simulink model "CompControl_V2"  (R2025b)
settings: Solver=ode45  StartTime=0.0  StopTime=t_f_cc  RelTol=1e-3
values from neighbouring files (symbols this model uses):
  dh_base = dh_raw    [CompControlTest_V2.m]    (also in NewRun.m)
  dq0_cc = zeros(length(joint_types), 1)    [CompControlTest_V2.m]    (also in NewRun.m = dq0)
  g0 = [0, 0, -9.81]    [CompControlTest_V2.m]    (also in EOMtestCode.m = [0 0 -9.81]; NewRun.m = input_ui.gValues; run.m = [0 0 -9.81]; test.m = input.g0)
  h_e = repmat(h_e', length(t), 1)    [CompControlTest_V2.m]    (also in NewRun.m)
  I_l = params.I_l(:)    [CompControlTest_V2.m]    (also in EOMtestCode.m = [IL1 IL2]; NewRun.m = I_l(:); run.m = sym('I_l', [N 1]); test.m = sym('I_l', [N 1]))
  I_m = params.I_m(:)    [CompControlTest_V2.m]    (also in EOMtestCode.m = [IM1 IM2]; NewRun.m = I_m(:); run.m = sym('I_m', [N 1]); test.m = sym('I_m', [N 1]))
  jt = zeros(N, 1)    [CompControlTest_V2.m]    (also in NewRun.m = zeros(DOF, 1))
  k_r = params.k_r(:)    [CompControlTest_V2.m]    (also in EOMtestCode.m = [kr1; kr2]; NewRun.m = k_r(:); run.m = sym('k_r', [N 1]); test.m = sym('k_r', [N 1]))
  KD = diag([ 45,  45,  45,  18,  18,  18])    [CompControlTest_V2.m]    (also in NewRun.m = eye(6)*K_d)
  KP = diag([500, 500, 500,  80,  80,  80])    [CompControlTest_V2.m]    (also in NewRun.m = eye(6)*K_p)
  m_l = params.m_l(:)    [CompControlTest_V2.m]    (also in EOMtestCode.m = [m1 m2]; NewRun.m = m_l(:); run.m = sym('m_l', [N 1]); test.m = sym('m_l', [N 1]))
  m_m = params.m_m(:)    [CompControlTest_V2.m]    (also in EOMtestCode.m = [mm1 mm2]; NewRun.m = m_m(:); run.m = sym('m_m', [N 1]); test.m = sym('m_m', [N 1]))
  q0_cc = zeros(length(joint_types), 1)    [CompControlTest_V2.m]    (also in NewRun.m = q0)
settings Model: Creator=ironc  LastModifiedBy=ironc

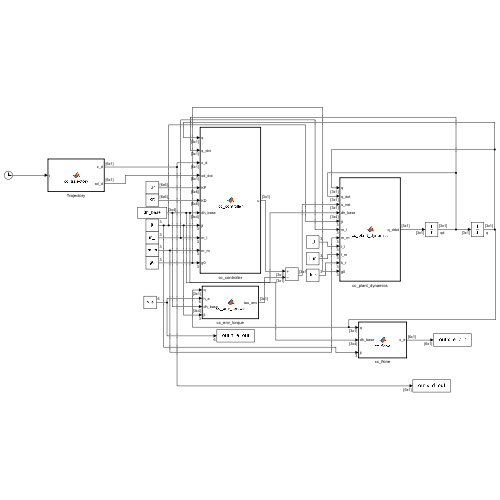
[thumbnail: Simulink's stored preview of the top-level diagram]
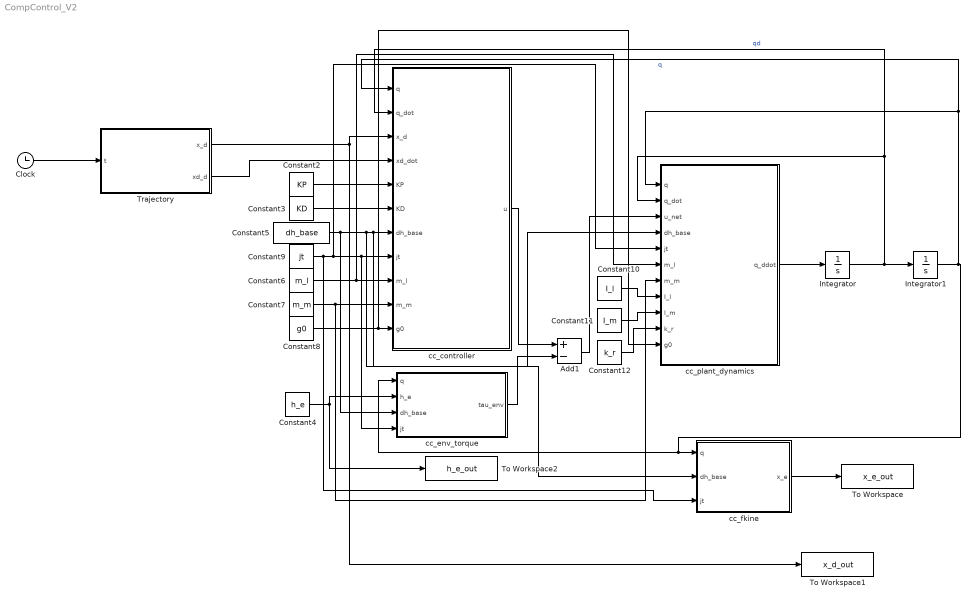
== system CompControl_V2 ==
  Add1 : Sum  Inputs=+-
  Clock : Clock
  Constant10 : Constant  Value=I_l
  Constant11 : Constant  Value=I_m
  Constant12 : Constant  Value=k_r
  Constant2 : Constant  Value=KP
  Constant3 : Constant  Value=KD
  Constant4 : Constant  Value=h_e
  Constant5 : Constant  Value=dh_base
  Constant6 : Constant  Value=m_l
  Constant7 : Constant  Value=m_m
  Constant8 : Constant  Value=g0
  Constant9 : Constant  Value=jt
  Integrator : Integrator  InitialCondition=dq0_cc
  Integrator1 : Integrator  InitialCondition=q0_cc
  To Workspace : ToWorkspace  VariableName=x_e_out  SaveFormat=Timeseries  SampleTime=-1
  To Workspace1 : ToWorkspace  VariableName=x_d_out  SaveFormat=Timeseries  SampleTime=-1
  To Workspace2 : ToWorkspace  VariableName=h_e_out  SaveFormat=Timeseries  SampleTime=-1
  Trajectory : MATLAB Function  TreatAsAtomicUnit=on
  cc_controller : MATLAB Function  TreatAsAtomicUnit=on
  cc_env_torque : MATLAB Function  TreatAsAtomicUnit=on
  cc_fkine : MATLAB Function  TreatAsAtomicUnit=on
  cc_plant_dynamics : MATLAB Function  TreatAsAtomicUnit=on
  wires:
  Integrator1/1 -> cc_fkine/1(q), cc_env_torque/1(q), cc_controller/1(q), cc_plant_dynamics/1(q)  "q"
  Integrator/1 -> cc_plant_dynamics/2(q_dot), cc_controller/2(q_dot), Integrator1/1  "qd"
  Trajectory/1(x_d) -> cc_controller/3(x_d), To Workspace1/1
  cc_plant_dynamics/1(q_ddot) -> Integrator/1
  cc_env_torque/1(tau_env) -> Add1/2
  Trajectory/2(xd_d) -> cc_controller/4(xd_dot)
  Constant2/1 -> cc_controller/5(KP)
  Constant3/1 -> cc_controller/6(KD)
  cc_controller/1(u) -> Add1/1
  Constant4/1 -> To Workspace2/1, cc_env_torque/2(h_e)
  Add1/1 -> cc_plant_dynamics/3(u_net)
  cc_fkine/1(x_e) -> To Workspace/1
  Constant5/1 -> cc_env_torque/3(dh_base), cc_plant_dynamics/4(dh_base), cc_fkine/2(dh_base), cc_controller/7(dh_base)
  Constant6/1 -> cc_plant_dynamics/6(m_l), cc_controller/9(m_l)
  Constant7/1 -> cc_plant_dynamics/7(m_m), cc_controller/10(m_m)
  Constant8/1 -> cc_plant_dynamics/11(g0), cc_controller/11(g0)
  Constant9/1 -> cc_fkine/3(jt), cc_plant_dynamics/5(jt), cc_env_torque/4(jt), cc_controller/8(jt)
  Constant10/1 -> cc_plant_dynamics/8(I_l)
  Constant11/1 -> cc_plant_dynamics/9(I_m)
  Constant12/1 -> cc_plant_dynamics/10(k_r)
  Clock/1 -> Trajectory/1(t)

== matlab function CompControl_V2/cc_controller ==
  data: q input; u output; q_dot input; x_d input; xd_dot input; KP input; KD input; dh_base input; jt input; m_l input; m_m input; g0 input
function u = cc_controller(q, q_dot, x_d, xd_dot, KP, KD, dh_base, jt, m_l, m_m, g0)
% CC_CONTROLLER  Operational space PD + gravity compensation (compliance control).
%
%   u = J_A^T(q) * [KP * x̃ + KD * ẋ̃] + G(q)
%
%   where:
%       x̃      = x_d - x_e              (6x1 pose error)
%       ẋ̃      = ẋ_d - J_A(q)*q̇         (6x1 velocity error)
%       G(q)   = gravity compensation    (n x 1)
%
%   h_e is NOT in this function — it enters only at the plant
%   summing junction as -J^T(q)*h_e.  This is what makes it INDIRECT
%   (compliance) force control.  At equilibrium (eq. 9.3):
%       x̃ = KP^-1 * h_A    →   KP^-1 is the compliance matrix
%
%   All matrices computed inline — no extrinsic, no codegen issues.
%
% INPUTS:
%   q       - (n x 1) joint positions
%   q_dot   - (n x 1) joint velocities
%   x_d     - (6 x 1) desired pose     [px;py;pz;roll;pitch;yaw]
%   xd_dot  - (6 x 1) desired pose rate (zeros for regulation)
%   KP      - (6 x 6) stiffness gain   (KP^-1 = compliance matrix)
%   KD      - (6 x 6) damping gain
%   dh_base - (n x 4) DH table
%   jt      - (n x 1) joint types: 1=revolute, 0=prismatic
%   m_l     - (n x 1) link masses (needed for gravity)
%   m_m     - (n x 1) motor masses (needed for gravity)
%   g0      - (1 x 3) gravity vector
%
% OUTPUT:
%   u       - (n x 1) joint torque command
%
% SIMULINK: MATLAB Function block — no extrinsic calls.
% -------------------------------------------------------------------------

% Current end-effector pose and analytical Jacobian
x_e = fkine_pose_num(q, dh_base, jt);            % 6 x 1
JA  = analytical_jacobian_num(q, dh_base, jt);   % 6 x n

% Errors in task space
x_tilde    = x_d - x_e;                           % 6 x 1  pose error
xdot_tilde = xd_dot - JA * q_dot;                 % 6 x 1  velocity error

% PD wrench in task space
task_wrench = KP * x_tilde + KD * xdot_tilde;     % 6 x 1

% Map to joint space via J_A^T
u_pd  = JA' * task_wrench;                        % n x 1

% Gravity compensation — cancels G in plant dynamics
G_vec = gravity_G_num(q, dh_base, jt, m_l, m_m, g0);  % n x 1

u = u_pd + G_vec;                                 % n x 1
end

function x_e = fkine_pose_num(q, dh_base, jt)
% FKINE_POSE_NUM  End-effector pose as a 6x1 vector.
%
% INPUTS:
%   q        - (n x 1) joint positions
%   dh_base  - (n x 4) DH table (zeros where q goes)
%   jt       - (n x 1) joint types: 1=revolute, 0=prismatic
%
% OUTPUT:
%   x_e      - (6 x 1) [px; py; pz; roll; pitch; yaw]
%              ZYX RPY convention (same as tr2rpy in Robotics Toolbox)
%
% Pure numeric — fully Simulink codegen compatible.

n   = numel(q);
T0i = fk_transforms_num(q, dh_base, jt);
T0n = T0i(:,:,n);           % end-effector transform

p = T0n(1:3, 4);            % position

% ZYX RPY extraction from rotation matrix R
R = T0n(1:3, 1:3);
pitch = atan2(-R(3,1), sqrt(R(1,1)^2 + R(2,1)^2));
roll  = atan2( R(3,2), R(3,3));
yaw   = atan2( R(2,1), R(1,1));

x_e = [p; roll; pitch; yaw];   % 6 x 1
end

function T = homo_trans_num(a, alpha, d, theta)
% HOMO_TRANS_NUM  4x4 homogeneous transform from one DH row.
%   Standard DH convention: (a, alpha, d, theta)
%   Pure numeric — fully Simulink codegen compatible.

ct = cos(theta);  st = sin(theta);
ca = cos(alpha);  sa = sin(alpha);

T = [ct, -st*ca,  st*sa,  a*ct;
     st,  ct*ca, -ct*sa,  a*st;
      0,     sa,     ca,     d;
      0,      0,      0,     1];
end

function T0i = fk_transforms_num(q, dh_base, jt)
% FK_TRANSFORMS_NUM  Compute all T_0^i transforms for an n-DOF robot.
%
% INPUTS:
%   q        - (n x 1) joint positions [rad or m]
%   dh_base  - (n x 4) DH table [a, alpha, d, theta] with zeros where q goes
%   jt       - (n x 1) joint types: 1 = revolute, 0 = prismatic
%
% OUTPUT:
%   T0i      - (4 x 4 x n) stack of cumulative transforms T_0^1 ... T_0^n
%
% Pure numeric — fully Simulink codegen compatible.

n   = numel(q);
T0i = zeros(4, 4, n);

for i = 1:n
    a     = dh_base(i, 1);
    alpha = dh_base(i, 2);
    d     = dh_base(i, 3);
    theta = dh_base(i, 4);

    % Substitute joint variable into correct DH parameter
    if jt(i) == 1        % revolute  — q adds to theta
        theta = theta + q(i);
    else                 % prismatic — q adds to d
        d = d + q(i);
    end

    Ti = homo_trans_num(a, alpha, d, theta);

    if i == 1
        T0i(:,:,i) = Ti;
    else
        T0i(:,:,i) = T0i(:,:,i-1) * Ti;
    end
end
end

function JA = analytical_jacobian_num(q, dh_base, jt)
% ANALYTICAL_JACOBIAN_NUM  Analytical Jacobian J_A(q) — 6 x n.
%
%   ẋ_e = J_A * q̇    where ẋ_e = [ṗ; φ̇]  (position + RPY angle rates)
%
%   Built from geometric J and T_A:
%       J_A = blkdiag(I3, T_A^-1) * J
%
%   ZYX RPY T_A  (ω = T_A * [roll_dot; pitch_dot; yaw_dot]):
%       T_A = [cos(yaw)*cos(pitch), -sin(yaw), 0]
%             [sin(yaw)*cos(pitch),  cos(yaw), 0]
%             [-sin(pitch),          0,        1]
%
%   T_A is singular at pitch = ±90°. pinv handles this gracefully.
%
% INPUTS:
%   q        - (n x 1) joint positions
%   dh_base  - (n x 4) DH table
%   jt       - (n x 1) joint types: 1=revolute, 0=prismatic
%
% OUTPUT:
%   JA       - (6 x n) analytical Jacobian
%
% Pure numeric — fully Simulink codegen compatible.

J   = geom_jacobian_num(q, dh_base, jt);       % 6 x n
x_e = fkine_pose_num(q, dh_base, jt);          % 6 x 1

pitch = x_e(5);
yaw   = x_e(6);

TA = [ cos(yaw)*cos(pitch), -sin(yaw),  0;
       sin(yaw)*cos(pitch),  cos(yaw),  0;
      -sin(pitch),            0,         1];

TA_inv = pinv(TA);             % robust to singularity at pitch = ±90°

JA         = J;
JA(4:6,:)  = TA_inv * J(4:6,:);   % only angular rows change
end

function G = gravity_G_num(q, dh_base, jt, m_l, m_m, g0)
% GRAVITY_G_NUM  Gravity torque vector G(q) — n x 1.
%
%   G = -sum_i [ m_l(i)*(g0'*Jp_Li)' + m_m(i)*(g0'*Jp_Mi)' ]
%
%   Sign convention matches EOM.m: EOM.G = -simplify(G_raw)
%   so the equation of motion is B*q̈ + C*q̇ + G = u
%
% INPUTS:
%   q        - (n x 1) joint positions
%   dh_base  - (n x 4) DH table
%   jt       - (n x 1) joint types: 1=revolute, 0=prismatic
%   m_l      - (n x 1) link masses
%   m_m      - (n x 1) motor masses
%   g0       - (1 x 3) gravity direction e.g. [0, 0, -9.81]
%
% OUTPUT:
%   G        - (n x 1) gravity torque vector
%
% Pure numeric — fully Simulink codegen compatible.

n     = numel(q);
T0i   = fk_transforms_num(q, dh_base, jt);
g_vec = g0(:);                 % ensure 3 x 1
G     = zeros(n, 1);

for i = 1:n
    % Link COM position
    if i == 1
        P_prev = [0; 0; 0];
    else
        P_prev = T0i(1:3, 4, i-1);
    end
    P_Li = (P_prev + T0i(1:3, 4, i)) / 2;

    % Motor position
    if i == 1
        P_mi = [0; 0; 0];
    else
        P_mi = T0i(1:3, 4, i-1);
    end

    % Linear Jacobian columns for link i
    Jp_L = zeros(3, n);
    Jp_M = zeros(3, n);

    for j = 1:i
        if j == 1
            z_j1 = [0; 0; 1];
            P_j1 = [0; 0; 0];
        else
            z_j1 = T0i(1:3, 3, j-1);
            P_j1 = T0i(1:3, 4, j-1);
        end
        if jt(j) == 1
            Jp_L(:,j) = cross(z_j1, P_Li - P_j1);
        else
            Jp_L(:,j) = z_j1;
        end
    end

    for j = 1:i-1
        if j == 1
            z_j1 = [0; 0; 1];
            P_j1 = [0; 0; 0];
        else
            z_j1 = T0i(1:3, 3, j-1);
            P_j1 = T0i(1:3, 4, j-1);
        end
        if jt(j) == 1
            Jp_M(:,j) = cross(z_j1, P_mi - P_j1);
        else
            Jp_M(:,j) = z_j1;
        end
    end

    % Accumulate (negative sign matches EOM.m convention)
    G = G - m_l(i) * (g_vec' * Jp_L)' ...
          - m_m(i) * (g_vec' * Jp_M)';
end
end

function J = geom_jacobian_num(q, dh_base, jt)
% GEOM_JACOBIAN_NUM  Geometric Jacobian J(q) at the end-effector — 6 x n.
%
%   ẋ = J * q̇    where ẋ = [v; ω]  (linear + angular velocity)
%
%   Uses the standard formula:
%     Revolute  j:  Jp_j = z_{j-1} x (p_n - p_{j-1})
%                   Jo_j = z_{j-1}
%     Prismatic j:  Jp_j = z_{j-1}
%                   Jo_j = 0
%
% INPUTS:
%   q        - (n x 1) joint positions
%   dh_base  - (n x 4) DH table
%   jt       - (n x 1) joint types: 1=revolute, 0=prismatic
%
% OUTPUT:
%   J        - (6 x n) geometric Jacobian
%
% Pure numeric — fully Simulink codegen compatible.

n   = numel(q);
T0i = fk_transforms_num(q, dh_base, jt);
p_n = T0i(1:3, 4, n);          % end-effector position

Jp = zeros(3, n);
Jo = zeros(3, n);

for j = 1:n
    if j == 1
        z_j1 = [0; 0; 1];      % base z-axis
        p_j1 = [0; 0; 0];      % base origin
    else
        z_j1 = T0i(1:3, 3, j-1);
        p_j1 = T0i(1:3, 4, j-1);
    end

    if jt(j) == 1              % revolute
        Jp(:,j) = cross(z_j1, p_n - p_j1);
        Jo(:,j) = z_j1;
    else                       % prismatic
        Jp(:,j) = z_j1;
        Jo(:,j) = [0; 0; 0];
    end
end

J = [Jp; Jo];                  % 6 x n
end

== matlab function CompControl_V2/cc_fkine ==
  data: q input; x_e output; dh_base input; jt input
function x_e = cc_fkine(q, dh_base, jt)
% CC_FKINE  End-effector pose — 6 x 1  [px; py; pz; roll; pitch; yaw].
%
%   Logging/scope block only — not in the feedback control loop.
%   Used to produce the desired-vs-actual position plots for the rubric.
%
% INPUTS:
%   q        - (n x 1) joint positions
%   dh_base  - (n x 4) DH table
%   jt       - (n x 1) joint types: 1=revolute, 0=prismatic
%
% OUTPUT:
%   x_e      - (6 x 1) [px; py; pz; roll; pitch; yaw]
%
% SIMULINK: MATLAB Function block — no extrinsic calls.
% -------------------------------------------------------------------------

x_e = fkine_pose_num(q, dh_base, jt);          % 6 x 1
end

function x_e = fkine_pose_num(q, dh_base, jt)
% FKINE_POSE_NUM  End-effector pose as a 6x1 vector.
%
% INPUTS:
%   q        - (n x 1) joint positions
%   dh_base  - (n x 4) DH table (zeros where q goes)
%   jt       - (n x 1) joint types: 1=revolute, 0=prismatic
%
% OUTPUT:
%   x_e      - (6 x 1) [px; py; pz; roll; pitch; yaw]
%              ZYX RPY convention (same as tr2rpy in Robotics Toolbox)
%
% Pure numeric — fully Simulink codegen compatible.

n   = numel(q);
T0i = fk_transforms_num(q, dh_base, jt);
T0n = T0i(:,:,n);           % end-effector transform

p = T0n(1:3, 4);            % position

% ZYX RPY extraction from rotation matrix R
R = T0n(1:3, 1:3);
pitch = atan2(-R(3,1), sqrt(R(1,1)^2 + R(2,1)^2));
roll  = atan2( R(3,2), R(3,3));
yaw   = atan2( R(2,1), R(1,1));

x_e = [p; roll; pitch; yaw];   % 6 x 1
end

function T0i = fk_transforms_num(q, dh_base, jt)
% FK_TRANSFORMS_NUM  Compute all T_0^i transforms for an n-DOF robot.
%
% INPUTS:
%   q        - (n x 1) joint positions [rad or m]
%   dh_base  - (n x 4) DH table [a, alpha, d, theta] with zeros where q goes
%   jt       - (n x 1) joint types: 1 = revolute, 0 = prismatic
%
% OUTPUT:
%   T0i      - (4 x 4 x n) stack of cumulative transforms T_0^1 ... T_0^n
%
% Pure numeric — fully Simulink codegen compatible.

n   = numel(q);
T0i = zeros(4, 4, n);

for i = 1:n
    a     = dh_base(i, 1);
    alpha = dh_base(i, 2);
    d     = dh_base(i, 3);
    theta = dh_base(i, 4);

    % Substitute joint variable into correct DH parameter
    if jt(i) == 1        % revolute  — q adds to theta
        theta = theta + q(i);
    else                 % prismatic — q adds to d
        d = d + q(i);
    end

    Ti = homo_trans_num(a, alpha, d, theta);

    if i == 1
        T0i(:,:,i) = Ti;
    else
        T0i(:,:,i) = T0i(:,:,i-1) * Ti;
    end
end
end

function T = homo_trans_num(a, alpha, d, theta)
% HOMO_TRANS_NUM  4x4 homogeneous transform from one DH row.
%   Standard DH convention: (a, alpha, d, theta)
%   Pure numeric — fully Simulink codegen compatible.

ct = cos(theta);  st = sin(theta);
ca = cos(alpha);  sa = sin(alpha);

T = [ct, -st*ca,  st*sa,  a*ct;
     st,  ct*ca, -ct*sa,  a*st;
      0,     sa,     ca,     d;
      0,      0,      0,     1];
end

== matlab function CompControl_V2/cc_env_torque ==
  data: q input; tau_env output; h_e input; dh_base input; jt input
function tau_env = cc_env_torque(q, h_e, dh_base, jt)
% CC_ENV_TORQUE  Joint torque disturbance from end-effector contact force.
%
%   tau_env = J^T(q) * h_e          (right-hand side of eq. 9.1)
%
%   This is SUBTRACTED at the plant summing junction:
%       u_net = u_controller - tau_env
%
%   Uses the GEOMETRIC Jacobian J (not J_A).
%   The plant dynamics use J; the controller uses J_A.
%   h_e never enters the controller — indirect/compliance force control.
%
% INPUTS:
%   q        - (n x 1) joint positions
%   h_e      - (6 x 1) contact wrench [fx;fy;fz;mx;my;mz]  (N, N·m)
%   dh_base  - (n x 4) DH table
%   jt       - (n x 1) joint types: 1=revolute, 0=prismatic
%
% OUTPUT:
%   tau_env  - (n x 1) equivalent joint disturbance torques
%
% SIMULINK: MATLAB Function block — no extrinsic calls.
% -------------------------------------------------------------------------

J       = geom_jacobian_num(q, dh_base, jt);   % 6 x n  geometric Jacobian
tau_env = J' * h_e;                             % n x 1
end

function J = geom_jacobian_num(q, dh_base, jt)
% GEOM_JACOBIAN_NUM  Geometric Jacobian J(q) at the end-effector — 6 x n.
%
%   ẋ = J * q̇    where ẋ = [v; ω]  (linear + angular velocity)
%
%   Uses the standard formula:
%     Revolute  j:  Jp_j = z_{j-1} x (p_n - p_{j-1})
%                   Jo_j = z_{j-1}
%     Prismatic j:  Jp_j = z_{j-1}
%                   Jo_j = 0
%
% INPUTS:
%   q        - (n x 1) joint positions
%   dh_base  - (n x 4) DH table
%   jt       - (n x 1) joint types: 1=revolute, 0=prismatic
%
% OUTPUT:
%   J        - (6 x n) geometric Jacobian
%
% Pure numeric — fully Simulink codegen compatible.

n   = numel(q);
T0i = fk_transforms_num(q, dh_base, jt);
p_n = T0i(1:3, 4, n);          % end-effector position

Jp = zeros(3, n);
Jo = zeros(3, n);

for j = 1:n
    if j == 1
        z_j1 = [0; 0; 1];      % base z-axis
        p_j1 = [0; 0; 0];      % base origin
    else
        z_j1 = T0i(1:3, 3, j-1);
        p_j1 = T0i(1:3, 4, j-1);
    end

    if jt(j) == 1              % revolute
        Jp(:,j) = cross(z_j1, p_n - p_j1);
        Jo(:,j) = z_j1;
    else                       % prismatic
        Jp(:,j) = z_j1;
        Jo(:,j) = [0; 0; 0];
    end
end

J = [Jp; Jo];                  % 6 x n
end

function T0i = fk_transforms_num(q, dh_base, jt)
% FK_TRANSFORMS_NUM  Compute all T_0^i transforms for an n-DOF robot.
%
% INPUTS:
%   q        - (n x 1) joint positions [rad or m]
%   dh_base  - (n x 4) DH table [a, alpha, d, theta] with zeros where q goes
%   jt       - (n x 1) joint types: 1 = revolute, 0 = prismatic
%
% OUTPUT:
%   T0i      - (4 x 4 x n) stack of cumulative transforms T_0^1 ... T_0^n
%
% Pure numeric — fully Simulink codegen compatible.

n   = numel(q);
T0i = zeros(4, 4, n);

for i = 1:n
    a     = dh_base(i, 1);
    alpha = dh_base(i, 2);
    d     = dh_base(i, 3);
    theta = dh_base(i, 4);

    % Substitute joint variable into correct DH parameter
    if jt(i) == 1        % revolute  — q adds to theta
        theta = theta + q(i);
    else                 % prismatic — q adds to d
        d = d + q(i);
    end

    Ti = homo_trans_num(a, alpha, d, theta);

    if i == 1
        T0i(:,:,i) = Ti;
    else
        T0i(:,:,i) = T0i(:,:,i-1) * Ti;
    end
end
end

function T = homo_trans_num(a, alpha, d, theta)
% HOMO_TRANS_NUM  4x4 homogeneous transform from one DH row.
%   Standard DH convention: (a, alpha, d, theta)
%   Pure numeric — fully Simulink codegen compatible.

ct = cos(theta);  st = sin(theta);
ca = cos(alpha);  sa = sin(alpha);

T = [ct, -st*ca,  st*sa,  a*ct;
     st,  ct*ca, -ct*sa,  a*st;
      0,     sa,     ca,     d;
      0,      0,      0,     1];
end

== matlab function CompControl_V2/cc_plant_dynamics ==
  data: q input; q_ddot output; q_dot input; u_net input; dh_base input; jt input; m_l input; m_m input; I_l input; I_m input; k_r input; g0 input
function q_ddot = cc_plant_dynamics(q, q_dot, u_net, dh_base, jt, m_l, m_m, I_l, I_m, k_r, g0)
% CC_PLANT_DYNAMICS  Robot forward dynamics — plant block (eq. 9.1).
%
%   B(q)*q̈ = u_net - C(q,q̇)*q̇ - G(q)
%
%   u_net is the net torque AFTER the Simulink summing junction:
%       u_net = u_controller - J^T(q)*h_e
%
%   All matrices computed inline from DH parameters — no extrinsic calls,
%   no auto-generated files, no codegen issues.
%
% INPUTS:
%   q       - (n x 1) joint positions          [rad or m]
%   q_dot   - (n x 1) joint velocities         [rad/s or m/s]
%   u_net   - (n x 1) net torque = u - tau_env [N·m or N]
%   dh_base - (n x 4) DH table (zeros where q goes): [a, alpha, d, theta]
%   jt      - (n x 1) joint types: 1=revolute, 0=prismatic
%   m_l     - (n x 1) link masses [kg]
%   m_m     - (n x 1) motor masses [kg]
%   I_l     - (n x 1) link scalar inertias [kg·m²]
%   I_m     - (n x 1) motor scalar inertias [kg·m²]
%   k_r     - (n x 1) gear ratios [-]
%   g0      - (1 x 3) gravity vector e.g. [0, 0, -9.81]
%
% OUTPUT:
%   q_ddot  - (n x 1) joint accelerations [rad/s² or m/s²]
%              Feeds into the double integrator chain: q̈ → q̇ → q
%
% SIMULINK: MATLAB Function block
%   No extrinsic calls. All math is pure numeric MATLAB.
% -------------------------------------------------------------------------

B_mat  = inertia_B_num(q, dh_base, jt, m_l, m_m, I_l, I_m, k_r);
C_mat  = coriolis_C_num(q, q_dot, dh_base, jt, m_l, m_m, I_l, I_m, k_r);
G_vec  = gravity_G_num(q, dh_base, jt, m_l, m_m, g0);

% Backslash avoids explicit inv(B) — numerically stable since B is SPD
q_ddot = B_mat \ (u_net - C_mat * q_dot - G_vec);
end

function B = inertia_B_num(q, dh_base, jt, m_l, m_m, I_l, I_m, k_r)
% INERTIA_B_NUM  Mass/inertia matrix B(q) — n x n.
%
%   Computed from link and motor Jacobians following the same method
%   as EOM.m, but numerically at runtime instead of symbolically.
%
%   B = sum_i [ m_l(i)*Jp_L'*Jp_L + Jo_L'*R*Il*R'*Jo_L
%             + m_m(i)*Jp_M'*Jp_M + Jo_M'*Rmi*Im*Rmi'*Jo_M ]
%
%   I_l and I_m are treated as scalar (isotropic) link/motor inertias,
%   matching the EOM.m convention: I*eye(3).
%
% INPUTS:
%   q        - (n x 1) joint positions
%   dh_base  - (n x 4) DH table
%   jt       - (n x 1) joint types: 1=revolute, 0=prismatic
%   m_l      - (n x 1) link masses
%   m_m      - (n x 1) motor masses
%   I_l      - (n x 1) link scalar inertias
%   I_m      - (n x 1) motor scalar inertias
%   k_r      - (n x 1) gear ratios
%
% OUTPUT:
%   B        - (n x n) symmetric positive-definite inertia matrix
%
% Pure numeric — fully Simulink codegen compatible.

n   = numel(q);
T0i = fk_transforms_num(q, dh_base, jt);
B   = zeros(n, n);

for i = 1:n
    % ── Link COM position (midpoint of link i) ──────────────────────────
    if i == 1
        P_prev = [0; 0; 0];
    else
        P_prev = T0i(1:3, 4, i-1);
    end
    P_Li = (P_prev + T0i(1:3, 4, i)) / 2;

    % ── Motor position (at joint i origin) ──────────────────────────────
    if i == 1
        P_mi = [0; 0; 0];
    else
        P_mi = T0i(1:3, 4, i-1);
    end

    % ── Motor z-axis ─────────────────────────────────────────────────────
    if i == 1
        z_mi = [0; 0; 1];
    else
        z_mi = T0i(1:3, 3, i-1);
    end

    % ── Per-link Jacobians (3 x n each) ──────────────────────────────────
    Jp_L = zeros(3, n);
    Jo_L = zeros(3, n);
    Jp_M = zeros(3, n);
    Jo_M = zeros(3, n);

    for j = 1:i
        if j == 1
            z_j1 = [0; 0; 1];
            P_j1 = [0; 0; 0];
        else
            z_j1 = T0i(1:3, 3, j-1);
            P_j1 = T0i(1:3, 4, j-1);
        end

        if jt(j) == 1                          % revolute
            Jp_L(:,j) = cross(z_j1, P_Li - P_j1);
            Jo_L(:,j) = z_j1;
        else                                   % prismatic
            Jp_L(:,j) = z_j1;
            Jo_L(:,j) = [0; 0; 0];
        end

        % Motor angular Jacobian
        if j == i
            Jo_M(:,j) = k_r(i) * z_mi;
        else
            Jo_M(:,j) = Jo_L(:,j);
        end
    end

    for j = 1:i-1
        if j == 1
            z_j1 = [0; 0; 1];
            P_j1 = [0; 0; 0];
        else
            z_j1 = T0i(1:3, 3, j-1);
            P_j1 = T0i(1:3, 4, j-1);
        end

        if jt(j) == 1                          % revolute
            Jp_M(:,j) = cross(z_j1, P_mi - P_j1);
        else                                   % prismatic
            Jp_M(:,j) = z_j1;
        end
    end

    % ── Rotation matrices ─────────────────────────────────────────────────
    R_0i  = T0i(1:3, 1:3, i);
    if i == 1
        R_0mi = eye(3);
    else
        R_0mi = T0i(1:3, 1:3, i-1);
    end

    Il_mat = I_l(i) * eye(3);     % scalar inertia → isotropic 3x3
    Im_mat = I_m(i) * eye(3);

    % ── Accumulate B ──────────────────────────────────────────────────────
    B = B + m_l(i) * (Jp_L' * Jp_L) ...
          + Jo_L' * R_0i * Il_mat * R_0i' * Jo_L ...
          + m_m(i) * (Jp_M' * Jp_M) ...
          + Jo_M' * R_0mi * Im_mat * R_0mi' * Jo_M;
end
end

function T0i = fk_transforms_num(q, dh_base, jt)
% FK_TRANSFORMS_NUM  Compute all T_0^i transforms for an n-DOF robot.
%
% INPUTS:
%   q        - (n x 1) joint positions [rad or m]
%   dh_base  - (n x 4) DH table [a, alpha, d, theta] with zeros where q goes
%   jt       - (n x 1) joint types: 1 = revolute, 0 = prismatic
%
% OUTPUT:
%   T0i      - (4 x 4 x n) stack of cumulative transforms T_0^1 ... T_0^n
%
% Pure numeric — fully Simulink codegen compatible.

n   = numel(q);
T0i = zeros(4, 4, n);

for i = 1:n
    a     = dh_base(i, 1);
    alpha = dh_base(i, 2);
    d     = dh_base(i, 3);
    theta = dh_base(i, 4);

    % Substitute joint variable into correct DH parameter
    if jt(i) == 1        % revolute  — q adds to theta
        theta = theta + q(i);
    else                 % prismatic — q adds to d
        d = d + q(i);
    end

    Ti = homo_trans_num(a, alpha, d, theta);

    if i == 1
        T0i(:,:,i) = Ti;
    else
        T0i(:,:,i) = T0i(:,:,i-1) * Ti;
    end
end
end

function T = homo_trans_num(a, alpha, d, theta)
% HOMO_TRANS_NUM  4x4 homogeneous transform from one DH row.
%   Standard DH convention: (a, alpha, d, theta)
%   Pure numeric — fully Simulink codegen compatible.

ct = cos(theta);  st = sin(theta);
ca = cos(alpha);  sa = sin(alpha);

T = [ct, -st*ca,  st*sa,  a*ct;
     st,  ct*ca, -ct*sa,  a*st;
      0,     sa,     ca,     d;
      0,      0,      0,     1];
end

function C = coriolis_C_num(q, q_dot, dh_base, jt, m_l, m_m, I_l, I_m, k_r)
% CORIOLIS_C_NUM  Coriolis/centripetal matrix C(q, q̇) — n x n.
%
%   Computed from Christoffel symbols using numerical finite differences on B:
%
%     C(k,j) = sum_i  Gamma_kji * q̇_i
%
%     Gamma_kji = 0.5 * [ dB(k,j)/dq_i
%                        + dB(k,i)/dq_j
%                        - dB(i,j)/dq_k ]
%
%   dB/dq_i approximated by central finite differences on inertia_B_num.
%   This matches the symbolic Christoffel formula used in EOM.m.
%
% INPUTS:
%   q        - (n x 1) joint positions
%   q_dot    - (n x 1) joint velocities
%   dh_base  - (n x 4) DH table
%   jt       - (n x 1) joint types: 1=revolute, 0=prismatic
%   m_l, m_m - (n x 1) link/motor masses
%   I_l, I_m - (n x 1) link/motor scalar inertias
%   k_r      - (n x 1) gear ratios
%
% OUTPUT:
%   C        - (n x n) Coriolis/centripetal matrix
%
% Pure numeric — fully Simulink codegen compatible.

n   = numel(q);
eps = 1e-6;

% ── Step 1: compute dB/dq_i via central differences ─────────────────────
%   dB(:,:,i) = partial derivative of B with respect to q_i
dB = zeros(n, n, n);

for i = 1:n
    e_i        = zeros(n, 1);
    e_i(i)     = 1;
    B_plus     = inertia_B_num(q + eps*e_i, dh_base, jt, m_l, m_m, I_l, I_m, k_r);
    B_minus    = inertia_B_num(q - eps*e_i, dh_base, jt, m_l, m_m, I_l, I_m, k_r);
    dB(:,:,i)  = (B_plus - B_minus) / (2*eps);
end

% ── Step 2: assemble C from Christoffel symbols ──────────────────────────
C = zeros(n, n);

for k = 1:n
    for j = 1:n
        for i = 1:n
            C(k,j) = C(k,j) + 0.5 * ( dB(k,j,i) ...
                                      + dB(k,i,j) ...
                                      - dB(i,j,k) ) * q_dot(i);
        end
    end
end
end

function G = gravity_G_num(q, dh_base, jt, m_l, m_m, g0)
% GRAVITY_G_NUM  Gravity torque vector G(q) — n x 1.
%
%   G = -sum_i [ m_l(i)*(g0'*Jp_Li)' + m_m(i)*(g0'*Jp_Mi)' ]
%
%   Sign convention matches EOM.m: EOM.G = -simplify(G_raw)
%   so the equation of motion is B*q̈ + C*q̇ + G = u
%
% INPUTS:
%   q        - (n x 1) joint positions
%   dh_base  - (n x 4) DH table
%   jt       - (n x 1) joint types: 1=revolute, 0=prismatic
%   m_l      - (n x 1) link masses
%   m_m      - (n x 1) motor masses
%   g0       - (1 x 3) gravity direction e.g. [0, 0, -9.81]
%
% OUTPUT:
%   G        - (n x 1) gravity torque vector
%
% Pure numeric — fully Simulink codegen compatible.

n     = numel(q);
T0i   = fk_transforms_num(q, dh_base, jt);
g_vec = g0(:);                 % ensure 3 x 1
G     = zeros(n, 1);

for i = 1:n
    % Link COM position
    if i == 1
        P_prev = [0; 0; 0];
    else
        P_prev = T0i(1:3, 4, i-1);
    end
    P_Li = (P_prev + T0i(1:3, 4, i)) / 2;

    % Motor position
    if i == 1
        P_mi = [0; 0; 0];
    else
        P_mi = T0i(1:3, 4, i-1);
    end

    % Linear Jacobian columns for link i
    Jp_L = zeros(3, n);
    Jp_M = zeros(3, n);

    for j = 1:i
        if j == 1
            z_j1 = [0; 0; 1];
            P_j1 = [0; 0; 0];
        else
            z_j1 = T0i(1:3, 3, j-1);
            P_j1 = T0i(1:3, 4, j-1);
        end
        if jt(j) == 1
            Jp_L(:,j) = cross(z_j1, P_Li - P_j1);
        else
            Jp_L(:,j) = z_j1;
        end
    end

    for j = 1:i-1
        if j == 1
            z_j1 = [0; 0; 1];
            P_j1 = [0; 0; 0];
        else
            z_j1 = T0i(1:3, 3, j-1);
            P_j1 = T0i(1:3, 4, j-1);
        end
        if jt(j) == 1
            Jp_M(:,j) = cross(z_j1, P_mi - P_j1);
        else
            Jp_M(:,j) = z_j1;
        end
    end

    % Accumulate (negative sign matches EOM.m convention)
    G = G - m_l(i) * (g_vec' * Jp_L)' ...
          - m_m(i) * (g_vec' * Jp_M)';
end
end

== matlab function CompControl_V2/Trajectory ==
  data: t input; x_d output; xd_d output
function [x_d, xd_d] = cc_trajectory(t)
% CC_TRAJECTORY  Simulink MATLAB Function block — trajectory evaluator.
%
%   Calls the function handles x_d(t) and xd_d(t) that are defined
%   in the run script and stored in the base workspace.
%
%
% INPUT:
%   t     - (1x1) current time  <-- wire from Clock block
%
% OUTPUTS:
%   x_d   - (6x1) desired pose      --> cc_controller x_d port
%   xd_d  - (6x1) desired pose rate --> cc_controller xd_dot port
%
% SIMULINK: MATLAB Function block
%   No Constant blocks needed for x_d or xd_d — just a Clock block.
% -------------------------------------------------------------------------
 
% Mark eval_trajectory as extrinsic so Simulink runs it interpreted.
% This allows evalin() inside it to reach the base workspace handles.
coder.extrinsic('eval_trajectory');
 
% Pre-declare output sizes (required for Simulink port size inference)
x_d  = zeros(6, 1);
xd_d = zeros(6, 1);
 
% Call the extrinsic wrapper — retrieves and evaluates the handles
[x_d, xd_d] = eval_trajectory(t);
end
